simulink library "Enrg_conv_El_to_Mec_Bosch"  (R2016a)
settings: Solver=ode1  StartTime=0.0  StopTime=Inf  FixedStep=0.001  RelTol=1e-3
undefined symbols (not defined in the file): drvEmot_RefTqeMOT, FirstDrivenAxle_FirstDrivenAxleNoOfEmot, FMIKit, SecondDrivenAxle_SecondDrivenAxleNoOfEmot
libraries: Enrg_conv_El_to_Mec_Bosch x13, Electrical_converter x8
(part 5 of 5)

== system Enrg_conv_El_to_Mec_Bosch/PTI_DriveEmot_Bosch_10ms/AWR2_3/ZeroWhenNotReady2 ==
  Bus Creator4 : BusCreator  Inputs=11
  zero_EMD3_ACT_DcLinkVoltage : Constant  Value=0
  zero_EMD4_ACT_DcLinkPower : Constant  Value=0
  zero_EMD4_ACT_DigitalInput1 : Constant  Value=0
  zero_EMD4_ACT_InverterState : Constant  Value=0
  zero_EMD4_ACT_MaxJunctionTemperature : Constant  Value=0
  zero_EMD4_ACT_MaximumAvailableTorque : Constant  Value=0
  zero_EMD4_ACT_MotorSpeed : Constant  Value=0
  zero_EMD4_ACT_MotorTemperature : Constant  Value=0
  zero_EMD4_ACT_MotorTorque : Constant  Value=0
  zero_EMD4_ACT_ReferenceTorqueLimited : Constant  Value=0
  zero_trqEmot1DesPhy : Constant  Value=0
  Out1 : Outport
  wires:
  zero_EMD4_ACT_MotorTemperature/1 -> Bus Creator4/11  "EMD_ACT_MotorTemperature"
  zero_EMD4_ACT_MaxJunctionTemperature/1 -> Bus Creator4/10  "EMD_ACT_MaxJunctionTemperature"
  zero_trqEmot1DesPhy/1 -> Bus Creator4/9  "trqEmotDesPhy"
  zero_EMD4_ACT_ReferenceTorqueLimited/1 -> Bus Creator4/8  "EMD_ACT_ReferenceTorqueLimited"
  zero_EMD4_ACT_InverterState/1 -> Bus Creator4/7  "EMD_ACT_InverterState"
  zero_EMD4_ACT_MotorTorque/1 -> Bus Creator4/6  "EMD_ACT_MotorTorque"
  zero_EMD4_ACT_MotorSpeed/1 -> Bus Creator4/5  "EMD_ACT_MotorSpeed"
  zero_EMD4_ACT_DcLinkPower/1 -> Bus Creator4/4  "EMD_ACT_DcLinkPower"
  zero_EMD4_ACT_MaximumAvailableTorque/1 -> Bus Creator4/3  "EMD_ACT_MaximumAvailableTorque"
  zero_EMD4_ACT_DigitalInput1/1 -> Bus Creator4/2  "EMD_ACT_DigitalInput1"
  zero_EMD3_ACT_DcLinkVoltage/1 -> Bus Creator4/1  "EMD3_ACT_DcLinkVoltage"
  Bus Creator4/1 -> Out1/1  "awr3B"

== system Enrg_conv_El_to_Mec_Bosch/PTI_DriveEmot_Bosch_10ms/EMD1_CMD_Command/Compare To Constant ==
  u : Inport
  Compare : RelationalOperator  Operator===  OutDataTypeStr=boolean  InputSameDT=on
  Constant : Constant  DisableCoverage=on  Value=const  OutDataTypeStr=Inherit: Inherit via back propagation
  y : Outport
  wires:
  u/1 -> Compare/1
  Constant/1 -> Compare/2
  Compare/1 -> y/1

== system Enrg_conv_El_to_Mec_Bosch/PTI_DriveEmot_Bosch_10ms/EMD1_CMD_Command/Compare To Constant1 ==
  u : Inport
  Compare : RelationalOperator  Operator===  OutDataTypeStr=boolean  InputSameDT=on
  Constant : Constant  DisableCoverage=on  Value=const  OutDataTypeStr=Inherit: Inherit via back propagation
  y : Outport
  wires:
  u/1 -> Compare/1
  Constant/1 -> Compare/2
  Compare/1 -> y/1

== system Enrg_conv_El_to_Mec_Bosch/PTI_DriveEmot_Bosch_10ms/EMD1_CMD_Command1/Compare To Constant ==
  u : Inport
  Compare : RelationalOperator  Operator===  OutDataTypeStr=boolean  InputSameDT=on
  Constant : Constant  DisableCoverage=on  Value=const  OutDataTypeStr=Inherit: Inherit via back propagation
  y : Outport
  wires:
  u/1 -> Compare/1
  Constant/1 -> Compare/2
  Compare/1 -> y/1

== system Enrg_conv_El_to_Mec_Bosch/PTI_DriveEmot_Bosch_10ms/EMD1_CMD_Command1/Compare To Constant1 ==
  u : Inport
  Compare : RelationalOperator  Operator===  OutDataTypeStr=boolean  InputSameDT=on
  Constant : Constant  DisableCoverage=on  Value=const  OutDataTypeStr=Inherit: Inherit via back propagation
  y : Outport
  wires:
  u/1 -> Compare/1
  Constant/1 -> Compare/2
  Compare/1 -> y/1

== system Enrg_conv_El_to_Mec_Bosch/PTI_DriveEmot_Bosch_10ms/EMD1_CMD_Command2/Compare To Constant ==
  u : Inport
  Compare : RelationalOperator  Operator===  OutDataTypeStr=boolean  InputSameDT=on
  Constant : Constant  DisableCoverage=on  Value=const  OutDataTypeStr=Inherit: Inherit via back propagation
  y : Outport
  wires:
  u/1 -> Compare/1
  Constant/1 -> Compare/2
  Compare/1 -> y/1

== system Enrg_conv_El_to_Mec_Bosch/PTI_DriveEmot_Bosch_10ms/EMD1_CMD_Command2/Compare To Constant1 ==
  u : Inport
  Compare : RelationalOperator  Operator===  OutDataTypeStr=boolean  InputSameDT=on
  Constant : Constant  DisableCoverage=on  Value=const  OutDataTypeStr=Inherit: Inherit via back propagation
  y : Outport
  wires:
  u/1 -> Compare/1
  Constant/1 -> Compare/2
  Compare/1 -> y/1

== system Enrg_conv_El_to_Mec_Bosch/PTI_DriveEmot_Bosch_10ms/EMD1_CMD_Command3/Compare To Constant ==
  u : Inport
  Compare : RelationalOperator  Operator===  OutDataTypeStr=boolean  InputSameDT=on
  Constant : Constant  DisableCoverage=on  Value=const  OutDataTypeStr=Inherit: Inherit via back propagation
  y : Outport
  wires:
  u/1 -> Compare/1
  Constant/1 -> Compare/2
  Compare/1 -> y/1

== system Enrg_conv_El_to_Mec_Bosch/PTI_DriveEmot_Bosch_10ms/EMD1_CMD_Command3/Compare To Constant1 ==
  u : Inport
  Compare : RelationalOperator  Operator===  OutDataTypeStr=boolean  InputSameDT=on
  Constant : Constant  DisableCoverage=on  Value=const  OutDataTypeStr=Inherit: Inherit via back propagation
  y : Outport
  wires:
  u/1 -> Compare/1
  Constant/1 -> Compare/2
  Compare/1 -> y/1

== matlab function Enrg_conv_El_to_Mec_Bosch/PTI_DriveEmot_Bosch/MotorSelection/Truth Table ==
  data: u1 input; y1 output; u2 input; y2 output; y3 output; y4 output
function [y1, y2, y3, y4] = fcn(u1, u2)

aVarTruthTableCondition_1 = false;
aVarTruthTableCondition_2 = false;
aVarTruthTableCondition_3 = false;
aVarTruthTableCondition_4 = false;
aVarTruthTableCondition_5 = false;
aVarTruthTableCondition_6 = false;
aVarTruthTableCondition_7 = false;
aVarTruthTableCondition_8 = false;
aVarTruthTableCondition_9 = false;


% 1stDrivenAxle - 0  and 2ndDrivenAxle - 0 [Not Valid]

aVarTruthTableCondition_1 = logical(u1 == 0 && u2 == 0);

% 1stDrivenAxle - 0  and 2ndDrivenAxle - 1 [Not Valid]

aVarTruthTableCondition_2 = logical(u1 == 0 && u2 == 1);

% 1stDrivenAxle - 0  and 2ndDrivenAxle - 2 [Not Valid]

aVarTruthTableCondition_3 = logical(u1 == 0 && u2 == 2);

% 1stDrivenAxle - 1  and 2ndDrivenAxle - 0 [Emot1,-]

aVarTruthTableCondition_4 = logical(u1 == 1 && u2 == 0);

% 1stDrivenAxle - 1  and 2ndDrivenAxle - 1 [Emot1, Emot3]

aVarTruthTableCondition_5 = logical(u1 == 1 && u2 == 1);

% 1stDrivenAxle - 1  and 2ndDrivenAxle - 2 [Emot1, Emot3+Emot4]

aVarTruthTableCondition_6 = logical(u1 == 1 && u2 == 2);

% 1stDrivenAxle - 2  and 2ndDrivenAxle - 0 [Emot1+Emot2,-]

aVarTruthTableCondition_7 = logical(u1 == 2 && u2 == 0);

% 1stDrivenAxle - 2  and 2ndDrivenAxle - 1 [Emot1+Emot2,Emot3]

aVarTruthTableCondition_8 = logical(u1 == 2 && u2 == 1);

% 1stDrivenAxle - 2  and2ndDrivenAxle - 2 [Emot1+Emot2,Emot3+Emot4]

aVarTruthTableCondition_9 = logical(u1 == 2 && u2 == 2);

if (aVarTruthTableCondition_1 && ~aVarTruthTableCondition_2 && ~aVarTruthTableCondition_3 && ~aVarTruthTableCondition_4 && ~aVarTruthTableCondition_5 && ~aVarTruthTableCondition_6 && ~aVarTruthTableCondition_7 && ~aVarTruthTableCondition_8 && ~aVarTruthTableCondition_9)
    aFcnTruthTableAction_1();
elseif (~aVarTruthTableCondition_1 && aVarTruthTableCondition_2 && ~aVarTruthTableCondition_3 && ~aVarTruthTableCondition_4 && ~aVarTruthTableCondition_5 && ~aVarTruthTableCondition_6 && ~aVarTruthTableCondition_7 && ~aVarTruthTableCondition_8 && ~aVarTruthTableCondition_9)
    aFcnTruthTableAction_2();
elseif (~aVarTruthTableCondition_1 && ~aVarTruthTableCondition_2 && aVarTruthTableCondition_3 && ~aVarTruthTableCondition_4 && ~aVarTruthTableCondition_5 && ~aVarTruthTableCondition_6 && ~aVarTruthTableCondition_7 && ~aVarTruthTableCondition_8 && ~aVarTruthTableCondition_9)
    aFcnTruthTableAction_3();
elseif (~aVarTruthTableCondition_1 && ~aVarTruthTableCondition_2 && ~aVarTruthTableCondition_3 && aVarTruthTableCondition_4 && ~aVarTruthTableCondition_5 && ~aVarTruthTableCondition_6 && ~aVarTruthTableCondition_7 && ~aVarTruthTableCondition_8 && ~aVarTruthTableCondition_9)
    aFcnTruthTableAction_4();
elseif (~aVarTruthTableCondition_1 && ~aVarTruthTableCondition_2 && ~aVarTruthTableCondition_3 && ~aVarTruthTableCondition_4 && aVarTruthTableCondition_5 && ~aVarTruthTableCondition_6 && ~aVarTruthTableCondition_7 && ~aVarTruthTableCondition_8 && ~aVarTruthTableCondition_9)
    aFcnTruthTableAction_5();
elseif (~aVarTruthTableCondition_1 && ~aVarTruthTableCondition_2 && ~aVarTruthTableCondition_3 && ~aVarTruthTableCondition_4 && ~aVarTruthTableCondition_5 && aVarTruthTableCondition_6 && ~aVarTruthTableCondition_7 && ~aVarTruthTableCondition_8 && ~aVarTruthTableCondition_9)
    aFcnTruthTableAction_6();
elseif (~aVarTruthTableCondition_1 && ~aVarTruthTableCondition_2 && ~aVarTruthTableCondition_3 && ~aVarTruthTableCondition_4 && ~aVarTruthTableCondition_5 && ~aVarTruthTableCondition_6 && aVarTruthTableCondition_7 && ~aVarTruthTableCondition_8 && ~aVarTruthTableCondition_9)
    aFcnTruthTableAction_7();
elseif (~aVarTruthTableCondition_1 && ~aVarTruthTableCondition_2 && ~aVarTruthTableCondition_3 && ~aVarTruthTableCondition_4 && ~aVarTruthTableCondition_5 && ~aVarTruthTableCondition_6 && ~aVarTruthTableCondition_7 && aVarTruthTableCondition_8 && ~aVarTruthTableCondition_9)
    aFcnTruthTableAction_8();
elseif (~aVarTruthTableCondition_1 && ~aVarTruthTableCondition_2 && ~aVarTruthTableCondition_3 && ~aVarTruthTableCondition_4 && ~aVarTruthTableCondition_5 && ~aVarTruthTableCondition_6 && ~aVarTruthTableCondition_7 && ~aVarTruthTableCondition_8 && aVarTruthTableCondition_9)
    aFcnTruthTableAction_9();
else % Default
    aFcnTruthTableAction_10();
end

function aFcnTruthTableAction_1()

% 1stDrivenAxle - 0 
% 2ndDrivenAxle - 0
% NOT VALID

y1 = 0;
y2 = 0;
y3 = 0;
y4 = 0;

function aFcnTruthTableAction_2()

% 1stDrivenAxle - 0 
% 2ndDrivenAxle - 1
% NOT VALID

y1 = 0;
y2 = 0;
y3 = 0;
y4 = 0;

function aFcnTruthTableAction_3()

% 1stDrivenAxle - 0 
% 2ndDrivenAxle - 2
% NOT VALID

y1 = 0;
y2 = 0;
y3 = 0;
y4 = 0;

function aFcnTruthTableAction_4()

% 1stDrivenAxle - 1 
% 2ndDrivenAxle - 0 [Emot1,-]

y1 = 1;
y2 = 0;
y3 = 0;
y4 = 0;

function aFcnTruthTableAction_5()

% 1stDrivenAxle - 1  
% 2ndDrivenAxle - 1 [Emot1, Emot3]

y1 = 1;
y2 = 0;
y3 = 1;
y4 = 0;

function aFcnTruthTableAction_6()

% 1stDrivenAxle - 1 
% 2ndDrivenAxle - 2 [Emot1, Emot3+Emot4]

y1 = 1;
y2 = 0;
y3 = 1;
y4 = 1;

function aFcnTruthTableAction_7()

% 1stDrivenAxle - 2  
% 2ndDrivenAxle - 0 [Emot1+Emot2,-]

y1 = 1;
y2 = 1;
y3 = 0;
y4 = 0;

function aFcnTruthTableAction_8()

% 1stDrivenAxle - 2  
% 2ndDrivenAxle - 1 [Emot1+Emot2,Emot3]

y1 = 1;
y2 = 1;
y3 = 1;
y4 = 0;

function aFcnTruthTableAction_9()

% 1stDrivenAxle - 2
% 2ndDrivenAxle - 2 [Emot1+Emot2,Emot3+Emot4]

y1 = 1;
y2 = 1;
y3 = 1;
y4 = 1;

function aFcnTruthTableAction_10()

% Default

y1 = 0;
y2 = 0;
y3 = 0;
y4 = 0;

== matlab function Enrg_conv_El_to_Mec_Bosch/PTI_DriveEmot_Bosch_10ms/MotorSelection/Truth Table ==
  data: u1 input; y1 output; u2 input; y2 output; y3 output; y4 output
function [y1, y2, y3, y4] = fcn(u1, u2)

aVarTruthTableCondition_1 = false;
aVarTruthTableCondition_2 = false;
aVarTruthTableCondition_3 = false;
aVarTruthTableCondition_4 = false;
aVarTruthTableCondition_5 = false;
aVarTruthTableCondition_6 = false;
aVarTruthTableCondition_7 = false;
aVarTruthTableCondition_8 = false;
aVarTruthTableCondition_9 = false;


% 1stDrivenAxle - 0  and 2ndDrivenAxle - 0 [Not Valid]

aVarTruthTableCondition_1 = logical(u1 == 0 && u2 == 0);

% 1stDrivenAxle - 0  and 2ndDrivenAxle - 1 [Not Valid]

aVarTruthTableCondition_2 = logical(u1 == 0 && u2 == 1);

% 1stDrivenAxle - 0  and 2ndDrivenAxle - 2 [Not Valid]

aVarTruthTableCondition_3 = logical(u1 == 0 && u2 == 2);

% 1stDrivenAxle - 1  and 2ndDrivenAxle - 0 [Emot1,-]

aVarTruthTableCondition_4 = logical(u1 == 1 && u2 == 0);

% 1stDrivenAxle - 1  and 2ndDrivenAxle - 1 [Emot1, Emot3]

aVarTruthTableCondition_5 = logical(u1 == 1 && u2 == 1);

% 1stDrivenAxle - 1  and 2ndDrivenAxle - 2 [Emot1, Emot3+Emot4]

aVarTruthTableCondition_6 = logical(u1 == 1 && u2 == 2);

% 1stDrivenAxle - 2  and 2ndDrivenAxle - 0 [Emot1+Emot2,-]

aVarTruthTableCondition_7 = logical(u1 == 2 && u2 == 0);

% 1stDrivenAxle - 2  and 2ndDrivenAxle - 1 [Emot1+Emot2,Emot3]

aVarTruthTableCondition_8 = logical(u1 == 2 && u2 == 1);

% 1stDrivenAxle - 2  and2ndDrivenAxle - 2 [Emot1+Emot2,Emot3+Emot4]

aVarTruthTableCondition_9 = logical(u1 == 2 && u2 == 2);

if (aVarTruthTableCondition_1 && ~aVarTruthTableCondition_2 && ~aVarTruthTableCondition_3 && ~aVarTruthTableCondition_4 && ~aVarTruthTableCondition_5 && ~aVarTruthTableCondition_6 && ~aVarTruthTableCondition_7 && ~aVarTruthTableCondition_8 && ~aVarTruthTableCondition_9)
    aFcnTruthTableAction_1();
elseif (~aVarTruthTableCondition_1 && aVarTruthTableCondition_2 && ~aVarTruthTableCondition_3 && ~aVarTruthTableCondition_4 && ~aVarTruthTableCondition_5 && ~aVarTruthTableCondition_6 && ~aVarTruthTableCondition_7 && ~aVarTruthTableCondition_8 && ~aVarTruthTableCondition_9)
    aFcnTruthTableAction_2();
elseif (~aVarTruthTableCondition_1 && ~aVarTruthTableCondition_2 && aVarTruthTableCondition_3 && ~aVarTruthTableCondition_4 && ~aVarTruthTableCondition_5 && ~aVarTruthTableCondition_6 && ~aVarTruthTableCondition_7 && ~aVarTruthTableCondition_8 && ~aVarTruthTableCondition_9)
    aFcnTruthTableAction_3();
elseif (~aVarTruthTableCondition_1 && ~aVarTruthTableCondition_2 && ~aVarTruthTableCondition_3 && aVarTruthTableCondition_4 && ~aVarTruthTableCondition_5 && ~aVarTruthTableCondition_6 && ~aVarTruthTableCondition_7 && ~aVarTruthTableCondition_8 && ~aVarTruthTableCondition_9)
    aFcnTruthTableAction_4();
elseif (~aVarTruthTableCondition_1 && ~aVarTruthTableCondition_2 && ~aVarTruthTableCondition_3 && ~aVarTruthTableCondition_4 && aVarTruthTableCondition_5 && ~aVarTruthTableCondition_6 && ~aVarTruthTableCondition_7 && ~aVarTruthTableCondition_8 && ~aVarTruthTableCondition_9)
    aFcnTruthTableAction_5();
elseif (~aVarTruthTableCondition_1 && ~aVarTruthTableCondition_2 && ~aVarTruthTableCondition_3 && ~aVarTruthTableCondition_4 && ~aVarTruthTableCondition_5 && aVarTruthTableCondition_6 && ~aVarTruthTableCondition_7 && ~aVarTruthTableCondition_8 && ~aVarTruthTableCondition_9)
    aFcnTruthTableAction_6();
elseif (~aVarTruthTableCondition_1 && ~aVarTruthTableCondition_2 && ~aVarTruthTableCondition_3 && ~aVarTruthTableCondition_4 && ~aVarTruthTableCondition_5 && ~aVarTruthTableCondition_6 && aVarTruthTableCondition_7 && ~aVarTruthTableCondition_8 && ~aVarTruthTableCondition_9)
    aFcnTruthTableAction_7();
elseif (~aVarTruthTableCondition_1 && ~aVarTruthTableCondition_2 && ~aVarTruthTableCondition_3 && ~aVarTruthTableCondition_4 && ~aVarTruthTableCondition_5 && ~aVarTruthTableCondition_6 && ~aVarTruthTableCondition_7 && aVarTruthTableCondition_8 && ~aVarTruthTableCondition_9)
    aFcnTruthTableAction_8();
elseif (~aVarTruthTableCondition_1 && ~aVarTruthTableCondition_2 && ~aVarTruthTableCondition_3 && ~aVarTruthTableCondition_4 && ~aVarTruthTableCondition_5 && ~aVarTruthTableCondition_6 && ~aVarTruthTableCondition_7 && ~aVarTruthTableCondition_8 && aVarTruthTableCondition_9)
    aFcnTruthTableAction_9();
else % Default
    aFcnTruthTableAction_10();
end

function aFcnTruthTableAction_1()

% 1stDrivenAxle - 0 
% 2ndDrivenAxle - 0
% NOT VALID

y1 = 0;
y2 = 0;
y3 = 0;
y4 = 0;

function aFcnTruthTableAction_2()

% 1stDrivenAxle - 0 
% 2ndDrivenAxle - 1
% NOT VALID

y1 = 0;
y2 = 0;
y3 = 0;
y4 = 0;

function aFcnTruthTableAction_3()

% 1stDrivenAxle - 0 
% 2ndDrivenAxle - 2
% NOT VALID

y1 = 0;
y2 = 0;
y3 = 0;
y4 = 0;

function aFcnTruthTableAction_4()

% 1stDrivenAxle - 1 
% 2ndDrivenAxle - 0 [Emot1,-]

y1 = 1;
y2 = 0;
y3 = 0;
y4 = 0;

function aFcnTruthTableAction_5()

% 1stDrivenAxle - 1  
% 2ndDrivenAxle - 1 [Emot1, Emot3]

y1 = 1;
y2 = 0;
y3 = 1;
y4 = 0;

function aFcnTruthTableAction_6()

% 1stDrivenAxle - 1 
% 2ndDrivenAxle - 2 [Emot1, Emot3+Emot4]

y1 = 1;
y2 = 0;
y3 = 1;
y4 = 1;

function aFcnTruthTableAction_7()

% 1stDrivenAxle - 2  
% 2ndDrivenAxle - 0 [Emot1+Emot2,-]

y1 = 1;
y2 = 1;
y3 = 0;
y4 = 0;

function aFcnTruthTableAction_8()

% 1stDrivenAxle - 2  
% 2ndDrivenAxle - 1 [Emot1+Emot2,Emot3]

y1 = 1;
y2 = 1;
y3 = 1;
y4 = 0;

function aFcnTruthTableAction_9()

% 1stDrivenAxle - 2
% 2ndDrivenAxle - 2 [Emot1+Emot2,Emot3+Emot4]

y1 = 1;
y2 = 1;
y3 = 1;
y4 = 1;

function aFcnTruthTableAction_10()

% Default

y1 = 0;
y2 = 0;
y3 = 0;
y4 = 0;
